simulink library "lib_transmission2"  (Simulink 4.1.1)
values from neighbouring files (symbols this model uses):
  logFlag = 1    [advSACompMaskInit.m]    (also in advSACompMaskInitR13.m)
undefined symbols (not defined in the file or in its folder): cyc_mph, fc_map_spd, fc_max_trq, fc_spd_scale, fc_trq_scale, fd_inertia, fd_loss, fd_ratio, gb_dnshift_load, gb_dnshift_spd, gb_gear_number_lookup, gb_gears_num, gb_inertia, gb_loss_const, gb_loss_input_spd_coeff, gb_loss_input_trq_coeff, gb_loss_output_spd_coeff, gb_loss_output_trq_coeff, gb_map_spd_out, gb_map_trq_in, gb_map_trq_out, gb_num_init, gb_ratio, gb_shift_delay, gb_spd_scale, gb_trq_scale, gb_upshift_load, gb_upshift_spd, htc_inertia, htc_k_adv, htc_k_adv_coast, htc_lockup, htc_lockup_load, htc_lockup_spd, htc_lu_gear_range, htc_max_coast_tr, htc_min_coast_tr, htc_pump_loss_spd, htc_pump_loss_trq_lockup, htc_pump_loss_trq_unlock, htc_sr, htc_sr_coast, htc_tr, htc_tr_coast, htc_unlock_spd, mc_map_spd, mc_max_trq, mc_overtrq_factor, mc_spd_scale, mc_trq_scale, tc_loss, tc_mc_to_fc_ratio, tx_eff_map, tx_map_spd, tx_map_trq, tx_pg_r, tx_pg_s, tx_speed_dep, vc_clutch_bool, vc_idle_spd ... (+2)
libraries: lib_controls x1, lib_etc x1, lib_controls2 x1, lib_transmission x1
(part 12 of 17)

== system lib_transmission2/Gearbox Control/Gearbox Control manual shift logic/manual shift logic/gearbox  control ==
  note: local GOTO blocks:
  gb_trq_out_r : Inport  Port=1  LatchInput=off
  gb_spd_out_r : Inport  Port=2  LatchInput=off
  prev. Pout/Pin : Inport  Port=3  LatchInput=off
  tires are at traction limit : Inport  Port=4  LatchInput=off
  Block NOTES : Subsystem
      settings: RTWFcnNameOpts=Auto  RTWFileNameOpts=Auto
      mask Display: disp('Block\nNOTES')
  Constant : Constant  Orientation=left  Value=1
  Fcn : Fcn  Expr=1/u
  Fcn1 : Fcn  Orientation=up  Expr=1/u
  Gain1 : Gain  Gain=-1  Multiplication=Element-wise(K.*u)  SaturateOnIntegerOverflow=on
  Product2 : Product  Inputs=*/  Multiplication=Element-wise(.*)  SaturateOnIntegerOverflow=on
  Product3 : Product  Inputs=2  Multiplication=Element-wise(.*)  SaturateOnIntegerOverflow=on
  Rate Limiter : RateLimiter  Orientation=left  RisingSlewLimit=1/(gb_shift_delay+eps)  FallingSlewLimit=-1/(gb_shift_delay+eps)
  Saturation : Saturate  UpperLimit=1  LowerLimit=0.2  LinearizeAsGain=on
  Saturation1 : Saturate  UpperLimit=gb_gears_num  LowerLimit=1  LinearizeAsGain=on
  Switch : Switch  Threshold=eps
  allow downshift? : Subsystem
      settings: RTWFcnNameOpts=Auto  RTWFileNameOpts=Auto
  current gear number : Sum  Inputs=++  SaturateOnIntegerOverflow=on
  delta gear number : Switch  Threshold=eps
  downshift  command : Subsystem
      settings: RTWFcnNameOpts=Auto  RTWFileNameOpts=Auto
  engine torque capability : Lookup  Orientation=left  InputValues=fc_map_spd*fc_spd_scale  OutputValues=fc_max_trq*fc_trq_scale+eps
  est eng trq : Sum  Inputs=++  SaturateOnIntegerOverflow=on
  gb_spd_in_r : Product  Inputs=2  Multiplication=Element-wise(.*)  SaturateOnIntegerOverflow=on
  gear ratio : Lookup  Orientation=left  InputValues=[1:length(gb_ratio)]  OutputValues=gb_ratio
  gear ratio1 : Lookup  InputValues=[1:length(gb_ratio)]  OutputValues=gb_ratio
  gearbox speed estimator : Subsystem
      settings: RTWFcnNameOpts=Auto  RTWFileNameOpts=Auto
  load=T/ (maxT at spd) : Saturate  UpperLimit=1  LowerLimit=0  LinearizeAsGain=on
  prev gear number : Memory  Orientation=left  X0=gb_num_init  InheritSampleTime=off
      settings: RTWStateStorageClass=Auto
  prev gear ratio : Memory  Orientation=left  X0=gb_ratio(gb_num_init)  InheritSampleTime=off
      settings: RTWStateStorageClass=Auto
  shifting1 : Subsystem
      settings: RTWFcnNameOpts=Auto  RTWFileNameOpts=Auto
  upshift  command : Subsystem
      settings: RTWFcnNameOpts=Auto  RTWFileNameOpts=Auto
  ~gb_trq_in_r : Product  Inputs=3  Multiplication=Element-wise(.*)  SaturateOnIntegerOverflow=on
  gear ratio2 : Outport  Port=1  InitialOutput=0
  shifting : Outport  Port=2  InitialOutput=0
  gear number : Outport  Port=3  InitialOutput=0
  wires:
  [acc_mech_trq_est] -> est eng trq/2
  shifting1/1(out_1) -> shifting/1
  gear ratio1/1 -> gear ratio2/1
  current gear number/1 -> Saturation1/1
  Saturation/1 -> Fcn/1
  prev. Pout/Pin/1 -> Saturation/1
  gb_trq_out_r/1 -> ~gb_trq_in_r/1
  upshift  command/1(command) -> delta gear number/1, delta gear number/2
  downshift  command/1(command) -> Gain1/1
  Fcn1/1 -> ~gb_trq_in_r/3
  engine torque capability/1 -> Product2/2
  Fcn/1 -> ~gb_trq_in_r/2
  Saturation1/1 -> prev gear number/1, gear ratio1/1, gear number/1, Rate Limiter/1, shifting1/1(gear number)
  prev gear number/1 -> allow downshift?/1(prev gearnum), upshift  command/1(prev gear number), downshift  command/1(prev gear number), current gear number/1
  Product2/1 -> load=T/ (maxT at spd)/1
  Constant/1 -> Switch/1
  tires are at traction limit/1 -> Switch/2
  Rate Limiter/1 -> gear ratio/1
  gb_spd_out_r/1 -> gb_spd_in_r/1
  gb_spd_in_r/1 -> gearbox speed estimator/1(gb_spd_in_r if no gear change)
  gear ratio/1 -> prev gear ratio/1
  prev gear ratio/1 -> gb_spd_in_r/2, Fcn1/1
  Gain1/1 -> Product3/2
  Product3/1 -> delta gear number/3
  allow downshift?/1(allow shift) -> Product3/1
  gearbox speed estimator/1(Out1) -> engine torque capability/1, downshift  command/3(engine speed), upshift  command/3(engine speed)
  ~gb_trq_in_r/1 -> est eng trq/1
  est eng trq/1 -> Product2/1
  load=T/ (maxT at spd)/1 -> Switch/3
  Switch/1 -> upshift  command/2(engine load), downshift  command/2(engine load)
  delta gear number/1 -> current gear number/2

== system lib_transmission2/Gearbox Control/automatic transmission gearbox and htc advanced lock-up logic for htc shift logic for gearbox/gearbox control for use w/ AT/Block NOTES ==
  note: Lock-up of the HTC occurs when it is supposed to for the current gear, AND
      | the transmission isn't shifting, AND
      | the lockup wouldn't precipitate an immediate downshift.
  note: This gearbox control block computes the current gear number given the gearbox's
      | req'd output torque and speed and an estimate its efficiency.  Upshifts occur, given a
      | certain engine speed,  when the estimated engine load falls below the upshift curve
      | in engine speed/load space, and downshifts likewise occur when estimated engine
      | load rises above the downshift curve.  Separate upshift and downshift curves are
      | defined for each gear.  An upshift may not be immediately followed by a downshift.
      | If the tires are about to slip, don't upshift unless the engine would be at max. speed.
      | Enforce this rule by setting the load to 1 when the tires are about to slip.

== system lib_transmission2/Gearbox Control/automatic transmission gearbox and htc advanced lock-up logic for htc shift logic for gearbox/gearbox control for use w/ AT/Speed Dependent Shifting ==
  note: storing shifting and gear ratio
      | information to workspace
  note: decel case
  note: accel case
  note: accel
      | case
  note: decel
      | case
  note: delta speed
  note: SPEED
      | DEPENDENT
      | SHIFT
      | SIGNAL
  "velocity required (limited) " : Inport  Port=1  LatchInput=off
  Look-Up Table (gear for downshift) : Lookup  InputValues="tx_spd_dep_dnshift(:,1)   % vector of speeds m/s"  OutputValues="tx_spd_dep_dnshift(:,2)  % gear number--must be step function"
  Look-Up Table (gear for upshift) : Lookup  InputValues="tx_spd_dep_upshift(:,1)   % vector of speeds in m/s"  OutputValues="tx_spd_dep_upshift(:,2)  % gear number--must be step function"
  Mux : Mux  Inputs=2
      settings: DisplayOption=none
  Mux2 : Mux  Inputs=2
      settings: DisplayOption=none
  New gear ratio : ToWorkspace  VariableName=new_gear_ratio  SampleTime=0  SaveFormat=Array
      settings: MaxDataPoints=50000
  Rounding Function : Rounding  Operator=round
  Rounding Function1 : Rounding  Operator=round
  Saturation4 : Saturate  UpperLimit=gb_gears_num  LowerLimit=1  LinearizeAsGain=on
  Saturation5 : Saturate  UpperLimit=gb_gears_num  LowerLimit=1  LinearizeAsGain=on
  "delta speed (\"+\" is acceleration)" : Sum  Inputs=-+  SaturateOnIntegerOverflow=on
  gear ratio6 : Lookup  InputValues=[1:length(gb_ratio)]  OutputValues=gb_ratio
  gear ratio8 : Lookup  InputValues=[1:length(gb_ratio)]  OutputValues=gb_ratio
  prev veh speed : Memory  X0=1  InheritSampleTime=off
      settings: RTWStateStorageClass=Auto
  shifting : Subsystem  AncestorBlock=lib_controls/SubSystem/shifting
      settings: RTWFcnNameOpts=Auto  RTWFileNameOpts=Auto
  shifting1 : Subsystem  AncestorBlock=lib_controls/SubSystem/shifting
      settings: RTWFcnNameOpts=Auto  RTWFileNameOpts=Auto
  switch for gear number : Switch  Threshold=eps
  switch for gear ratio and shifting (muxed) : Switch  Threshold=eps
  total fuel used (gal) : ToWorkspace  VariableName=neg_gear_num  SampleTime=0  SaveFormat=Array
      settings: MaxDataPoints=50000
  gear ratio and shifting : Outport  Orientation=up  Port=1
  gear number : Outport  Port=2
  wires:
  Rounding Function1/1 -> Saturation5/1
  Look-Up Table (gear for downshift)/1 -> Rounding Function1/1
  Rounding Function/1 -> Saturation4/1
  Look-Up Table (gear for upshift)/1 -> Rounding Function/1
  "delta speed (\"+\" is acceleration)"/1 -> switch for gear ratio and shifting (muxed)/2, switch for gear number/2
  switch for gear number/1 -> gear number/1
  switch for gear ratio and shifting (muxed)/1 -> gear ratio and shifting/1, New gear ratio/1
  Saturation4/1 -> gear ratio6/1, shifting1/1(gear number), switch for gear number/1
  shifting1/1(out_1) -> Mux/2
  gear ratio6/1 -> Mux/1
  Saturation5/1 -> shifting/1(gear number), gear ratio8/1, total fuel used (gal)/1, switch for gear number/3
  gear ratio8/1 -> Mux2/1
  shifting/1(out_1) -> Mux2/2
  Mux/1 -> switch for gear ratio and shifting (muxed)/1
  Mux2/1 -> switch for gear ratio and shifting (muxed)/3
  prev veh speed/1 -> "delta speed (\"+\" is acceleration)"/1
  "velocity required (limited) "/1 -> Look-Up Table (gear for upshift)/1, Look-Up Table (gear for downshift)/1, "delta speed (\"+\" is acceleration)"/2, prev veh speed/1

== system lib_transmission2/Gearbox Control/automatic transmission gearbox and htc advanced lock-up logic for htc shift logic for gearbox/gearbox control for use w/ AT/allow downshift? ==
  prev gearnum : Inport  Port=1  LatchInput=off
  Logical Operator : Logic  Operator=NOR  Inputs=2
  Memory : Memory  X0=1  InheritSampleTime=off
      settings: RTWStateStorageClass=Auto
  Memory1 : Memory  X0=1  InheritSampleTime=off
      settings: RTWStateStorageClass=Auto
  Relational Operator1 : RelationalOperator  Operator=>
  Relational Operator2 : RelationalOperator  Operator=>
  allow shift : Outport  Port=1  InitialOutput=0
  wires:
  Logical Operator/1 -> allow shift/1
  prev gearnum/1 -> Relational Operator1/1, Memory/1, Relational Operator2/1
  Relational Operator1/1 -> Logical Operator/1
  Memory/1 -> Relational Operator1/2, Memory1/1
  Memory1/1 -> Relational Operator2/2
  Relational Operator2/1 -> Logical Operator/2

== system lib_transmission2/Gearbox Control/automatic transmission gearbox and htc advanced lock-up logic for htc shift logic for gearbox/gearbox control for use w/ AT/downshift  command ==
  prev gear number : Inport  Port=1  LatchInput=off
  engine load : Inport  Port=2  LatchInput=off
  engine speed : Inport  Port=3  LatchInput=off
  Mux : Mux  Inputs=2
      settings: DisplayOption=none
  Relational Operator : RelationalOperator  Operator=>
  load fraction : Subsystem  mask(Gear Selector){spd=gb_dnshift_spd, load=gb_dnshift_load}
      mask prompts: spd "Speeds:"; load "Load Fractions:"
      mask help:
      | This block will perform a linear interplation (extrapolation outside of bounds) to determine the shift point load fraction associated with the current gear number and speed.
      |
      | The Speeds parameter should be defined as an array of vectors containing speeds for each gear number.  The Load Fractions parameter should be defined as a array of vectors containing load fractions indexed by the speeds in the Speeds parameter for each gear number.
      settings: RTWFcnNameOpts=Auto  RTWFileNameOpts=Auto
      mask Help:
      | Reference the base workspace variables - gb_**shift_spd and gb_**shift_load  where ** is either up for upshift conditions or dn for downshift conditions.
      | 
      | Or define the arrays as follows:
      | 
      | {[spd1 spd2 spd3 spd4]; [spd1 spd2 spd3 spd4]; ...}
      | 
      | {[load1 load2 load3 load4]; [load1 load2 load3 load4]; ...}
      | 
      | where each array contains one row for each gear in the gearbox.  Speeds should be defined in rad/s and loads as a decimal fraction.
  command : Outport  Port=1  InitialOutput=0
  wires:
  Relational Operator/1 -> command/1
  engine speed/1 -> Mux/2
  prev gear number/1 -> Mux/1
  engine load/1 -> Relational Operator/1
  Mux/1 -> load fraction/1(In1)
  load fraction/1(Out1) -> Relational Operator/2

== system lib_transmission2/Gearbox Control/automatic transmission gearbox and htc advanced lock-up logic for htc shift logic for gearbox/gearbox control for use w/ AT/downshift  command1 ==
  prev gear number : Inport  Port=1  LatchInput=off
  engine load : Inport  Port=2  LatchInput=off
  engine speed : Inport  Port=3  LatchInput=off
  Mux : Mux  Inputs=2
      settings: DisplayOption=none
  Relational Operator : RelationalOperator  Operator=>
  load fraction : Subsystem  mask(Gear Selector){spd=gb_dnshift_spd, load=gb_dnshift_load}
      mask prompts: spd "Speeds:"; load "Load Fractions:"
      mask help:
      | This block will perform a linear interplation (extrapolation outside of bounds) to determine the shift point load fraction associated with the current gear number and speed.
      |
      | The Speeds parameter should be defined as an array of vectors containing speeds for each gear number.  The Load Fractions parameter should be defined as a array of vectors containing load fractions indexed by the speeds in the Speeds parameter for each gear number.
      settings: RTWFcnNameOpts=Auto  RTWFileNameOpts=Auto
      mask Help:
      | Reference the base workspace variables - gb_**shift_spd and gb_**shift_load  where ** is either up for upshift conditions or dn for downshift conditions.
      | 
      | Or define the arrays as follows:
      | 
      | {[spd1 spd2 spd3 spd4]; [spd1 spd2 spd3 spd4]; ...}
      | 
      | {[load1 load2 load3 load4]; [load1 load2 load3 load4]; ...}
      | 
      | where each array contains one row for each gear in the gearbox.  Speeds should be defined in rad/s and loads as a decimal fraction.
  command : Outport  Port=1  InitialOutput=0
  wires:
  engine speed/1 -> Mux/2
  load fraction/1(Out1) -> Relational Operator/2
  Mux/1 -> load fraction/1(In1)
  engine load/1 -> Relational Operator/1
  prev gear number/1 -> Mux/1
  Relational Operator/1 -> command/1

== system lib_transmission2/Gearbox Control/automatic transmission gearbox and htc advanced lock-up logic for htc shift logic for gearbox/gearbox control for use w/ AT/est. engine trq and spd ==
  prev gear number : Inport  Port=1  LatchInput=off
  " prev eta_gb" : Inport  Port=2  LatchInput=off
  gb_trq_out_r : Inport  Port=3  LatchInput=off
  gb_spd_out_r : Inport  Port=4  LatchInput=off
  Block NOTES : Subsystem
      settings: RTWFcnNameOpts=Auto  RTWFileNameOpts=Auto
      mask Display: disp('Block\nNOTES')
  Constant2 : Constant  Orientation=left  Value=[1 1]
  Constant5 : Constant  Orientation=left  Value=0
  Demux : Demux  Outputs=2  BusSelectionMode=off
  K_adv : Subsystem
      settings: RTWFcnNameOpts=Auto  RTWFileNameOpts=Auto
  Logical Operator : Logic  Operator=AND  Inputs=2
  Logical Operator1 : Logic  Operator=NOT  Inputs=1
  Memory : Memory  X0=0  InheritSampleTime=off
      settings: RTWStateStorageClass=Auto
  Mux1 : Mux  Inputs=2
      settings: DisplayOption=none
  Mux2 : Mux  Inputs=2
      settings: DisplayOption=none
  Relational Operator1 : RelationalOperator  Operator=>
  SR Look-Up Table SR=wout/win : Lookup  InputValues=htc_k_adv  OutputValues=htc_sr
  Saturation1 : Saturate  UpperLimit=1  LowerLimit=0.7  LinearizeAsGain=on
  Saturation2 : Saturate  UpperLimit=inf  LowerLimit=0  LinearizeAsGain=on
  Switch : Switch  Threshold=eps
  TR Look-Up Table TR=Tout/Tin : Lookup  InputValues=htc_k_adv  OutputValues=htc_tr
  TR,SR : Mux  Inputs=2
      settings: DisplayOption=none
  est eng trq : Sum  Inputs=++  SaturateOnIntegerOverflow=on
  gear ratio1 : Lookup  InputValues=[1:length(gb_ratio)]  OutputValues=gb_ratio
  ~eng trq and spd : Product  Inputs=*/  Multiplication=Element-wise(.*)  SaturateOnIntegerOverflow=on
  ~gb_spd_in_r : Product  Inputs=2  Multiplication=Element-wise(.*)  SaturateOnIntegerOverflow=on
  ~gb_trq_in_r : Product  Inputs=//*  Multiplication=Element-wise(.*)  SaturateOnIntegerOverflow=on
  est eng trq (Nm) : Outport  Port=1
  est eng spd (rad/s) : Outport  Port=2
  gb_spd_in_est (rad/s)1 : Outport  Port=3
  wires:
  est eng trq/1 -> Mux1/1, Relational Operator1/1, Mux2/1
  ~gb_trq_in_r/1 -> est eng trq/1
  ~gb_spd_in_r/1 -> Mux2/2, gb_spd_in_est (rad/s)1/1, Mux1/2
  [acc_mech_trq_est] -> est eng trq/2
  SR Look-Up Table SR=wout/win/1 -> TR,SR/2
  TR Look-Up Table TR=Tout/Tin/1 -> TR,SR/1
  K_adv/1(K_adv) -> SR Look-Up Table SR=wout/win/1, TR Look-Up Table TR=Tout/Tin/1
  Mux2/1 -> K_adv/1("Req'd output trq and spd (Nm), (rad/s)")
  ~eng trq and spd/1 -> Demux/1
  Mux1/1 -> ~eng trq and spd/1
  [locked_up] -> Memory/1
  Logical Operator/1 -> Switch/2
  Logical Operator1/1 -> Logical Operator/2
  Memory/1 -> Logical Operator1/1
  Demux/1 -> est eng trq (Nm)/1
  prev gear number/1 -> gear ratio1/1
  Relational Operator1/1 -> Logical Operator/1
  Constant5/1 -> Relational Operator1/2
  Saturation2/1 -> est eng spd (rad/s)/1
  Demux/2 -> Saturation2/1
  Saturation1/1 -> ~gb_trq_in_r/2
  " prev eta_gb"/1 -> Saturation1/1
  Switch/1 -> ~eng trq and spd/2
  Constant2/1 -> Switch/3
  TR,SR/1 -> Switch/1
  gear ratio1/1 -> ~gb_spd_in_r/1, ~gb_trq_in_r/1
  gb_spd_out_r/1 -> ~gb_spd_in_r/2
  gb_trq_out_r/1 -> ~gb_trq_in_r/3

== system lib_transmission2/Gearbox Control/automatic transmission gearbox and htc advanced lock-up logic for htc shift logic for gearbox/gearbox control for use w/ AT/est. engine trq and spd assuming lockup ==
  new gear number : Inport  Port=1  LatchInput=off
  " prev eta_gb" : Inport  Port=2  LatchInput=off
  gb_trq_out_r : Inport  Port=3  LatchInput=off
  gb_spd_in_est : Inport  Port=4  LatchInput=off
  Block NOTES : Subsystem
      settings: RTWFcnNameOpts=Auto  RTWFileNameOpts=Auto
      mask Display: disp('Block\nNOTES')
  Memory : Memory  X0=gb_ratio(1)  InheritSampleTime=off
      settings: RTWStateStorageClass=Auto
  Saturation1 : Saturate  UpperLimit=1  LowerLimit=0.7  LinearizeAsGain=on
  Saturation2 : Saturate  UpperLimit=inf  LowerLimit=0  LinearizeAsGain=on
  est eng trq : Sum  Inputs=++  SaturateOnIntegerOverflow=on
  gear ratio1 : Lookup  InputValues=[1:length(gb_ratio)]  OutputValues=gb_ratio
  ~gb_spd_in_r : Product  Inputs=*/*  Multiplication=Element-wise(.*)  SaturateOnIntegerOverflow=on
  ~gb_trq_in_r : Product  Inputs=//*  Multiplication=Element-wise(.*)  SaturateOnIntegerOverflow=on
  est eng trq (Nm) : Outport  Port=1
  est eng spd (rad/s) : Outport  Port=2
  wires:
  ~gb_spd_in_r/1 -> Saturation2/1
  est eng trq/1 -> est eng trq (Nm)/1
  ~gb_trq_in_r/1 -> est eng trq/1
  [acc_mech_trq_est] -> est eng trq/2
  gb_spd_in_est/1 -> ~gb_spd_in_r/3
  Memory/1 -> ~gb_spd_in_r/2
  Saturation2/1 -> est eng spd (rad/s)/1
  new gear number/1 -> gear ratio1/1
  gb_trq_out_r/1 -> ~gb_trq_in_r/3
  gear ratio1/1 -> Memory/1, ~gb_spd_in_r/1, ~gb_trq_in_r/1
  " prev eta_gb"/1 -> Saturation1/1
  Saturation1/1 -> ~gb_trq_in_r/2

== system lib_transmission2/Gearbox Control/automatic transmission gearbox and htc advanced lock-up logic for htc shift logic for gearbox/gearbox control for use w/ AT/htc lockup logic ==
  engine load (%) : Inport  Port=1  LatchInput=off
  gear num : Inport  Port=2  LatchInput=off
  Constant1 : Constant  Orientation=left  Value=0.5
  Constant2 : Constant  Value=0
  Constant3 : Constant  Value=0
  Constant4 : Constant  Value=-1
  Logical Operator : Logic  Operator=NOR  Inputs=2
  Memory1 : Memory  Orientation=left  X0=1  InheritSampleTime=off
      settings: RTWStateStorageClass=Auto
  Memory2 : Memory  X0=1  InheritSampleTime=off
      settings: RTWStateStorageClass=Auto
  Memory3 : Memory  X0=1  InheritSampleTime=off
      settings: RTWStateStorageClass=Auto
  Relational Operator : RelationalOperator  Operator=>=
  Relational Operator1 : RelationalOperator  Operator=>
  Relational Operator2 : RelationalOperator  Operator=<
  Relational Operator3 : RelationalOperator  Operator=<
  Saturation1 : Saturate  UpperLimit=1  LowerLimit=0  LinearizeAsGain=on
  Switch{,1..3} (4 alike) : Switch  Threshold=0.5
  current lock/unlock  status : Sum  Inputs=++  SaturateOnIntegerOverflow=on
  lock-up in high gears : Lookup  InputValues=[1:length(htc_lockup)]  OutputValues=htc_lockup
  lock-up in this gear : Lookup  InputValues=htc_lockup_load  OutputValues=htc_lockup_spd
  lock/unlock  gear range : Lookup  InputValues=[1:length(htc_lockup)]  OutputValues=htc_lu_gear_range
  unlock in this gear : Lookup  InputValues=htc_lockup_load  OutputValues=htc_unlock_spd
  htc L/UL : Outport  Port=1
  wires:
  Constant1/1 -> Relational Operator/2, Relational Operator1/1
  gear num/1 -> lock-up in high gears/1, lock/unlock  gear range/1
  lock-up in high gears/1 -> Relational Operator/1
  Relational Operator/1 -> Switch/2, Switch/1
  Switch/1 -> htc L/UL/1, Memory1/1
  lock/unlock  gear range/1 -> Relational Operator1/2
  lock-up in this gear/1 -> Relational Operator2/1
  unlock in this gear/1 -> Relational Operator3/2
  Relational Operator1/1 -> Switch1/2
  Constant2/1 -> Switch1/1
  Switch1/1 -> Switch/3
  Saturation1/1 -> Switch1/3
  Relational Operator2/1 -> Logical Operator/1, Switch3/2, Switch3/1
  Relational Operator3/1 -> Logical Operator/2
  Logical Operator/1 -> Switch2/2
  Constant3/1 -> Switch2/3
  Switch3/1 -> Switch2/1
  Constant4/1 -> Switch3/3
  current lock/unlock  status/1 -> Saturation1/1
  Memory1/1 -> current lock/unlock  status/1
  Switch2/1 -> current lock/unlock  status/2
  Memory2/1 -> Relational Operator2/2, Relational Operator3/1
  Memory3/1 -> lock-up in this gear/1, unlock in this gear/1
  engine load (%)/1 -> Memory3/1
  [gb_trq_out_a] -> Memory2/1

== system lib_transmission2/Gearbox Control/automatic transmission gearbox and htc advanced lock-up logic for htc shift logic for gearbox/gearbox control for use w/ AT/shifting1 ==
  gear number : Inport  Port=1  LatchInput=off
  Constant : Constant  Value=gb_shift_delay-1e-6
  Relational Operator : RelationalOperator  Operator=<
  time since last shift : Subsystem
      settings: RTWFcnNameOpts=Auto  RTWFileNameOpts=Auto
      mask Display: disp('time since\nlast shift')
  out_1 : Outport  Port=1  InitialOutput=0
  wires:
  Relational Operator/1 -> out_1/1
  gear number/1 -> time since last shift/1(in_1)
  Constant/1 -> Relational Operator/2
  time since last shift/1(out_1) -> Relational Operator/1

== system lib_transmission2/Gearbox Control/automatic transmission gearbox and htc advanced lock-up logic for htc shift logic for gearbox/gearbox control for use w/ AT/upshift  command ==
  prev gear number : Inport  Port=1  LatchInput=off
  engine load : Inport  Port=2  LatchInput=off
  engine speed : Inport  Port=3  LatchInput=off
  Mux : Mux  Inputs=2
      settings: DisplayOption=none
  Relational Operator : RelationalOperator  Operator=<
  load fraction : Subsystem  mask(Gear Selector){spd=gb_upshift_spd, load=gb_upshift_load}
      mask prompts: spd "Speeds:"; load "Load Fractions:"
      mask help:
      | This block will perform a linear interplation (extrapolation outside of bounds) to determine the shift point load fraction associated with the current gear number and speed.
      |
      | The Speeds parameter should be defined as an array of vectors containing speeds for each gear number.  The Load Fractions parameter should be defined as a array of vectors containing load fractions indexed by the speeds in the Speeds parameter for each gear number.
      settings: RTWFcnNameOpts=Auto  RTWFileNameOpts=Auto
      mask Help:
      | Reference the base workspace variables - gb_**shift_spd and gb_**shift_load  where ** is either up for upshift conditions or dn for downshift conditions.
      | 
      | Or define the arrays as follows:
      | 
      | {[spd1 spd2 spd3 spd4]; [spd1 spd2 spd3 spd4]; ...}
      | 
      | {[load1 load2 load3 load4]; [load1 load2 load3 load4]; ...}
      | 
      | where each array contains one row for each gear in the gearbox.  Speeds should be defined in rad/s and loads as a decimal fraction.
  command : Outport  Port=1  InitialOutput=0
  wires:
  Relational Operator/1 -> command/1
  engine speed/1 -> Mux/2
  Mux/1 -> load fraction/1(In1)
  prev gear number/1 -> Mux/1
  engine load/1 -> Relational Operator/1
  load fraction/1(Out1) -> Relational Operator/2

== system lib_transmission2/Gearbox Control/automatic transmission gearbox and htc standard lockup logic for htc shift logic for gearbox/gearbox control for use w/ AT/Block NOTES ==
  note: This gearbox control block computes the current gear number given the gearbox's
      | req'd output torque and speed and an estimate its efficiency.  Upshifts occur, given a
      | certain engine speed,  when the estimated engine load falls below the upshift curve
      | in engine speed/load space, and downshifts likewise occur when estimated engine
      | load rises above the downshift curve.  Separate upshift and downshift curves are
      | defined for each gear.  An upshift may not be immediately followed by a downshift.
      | If the tires are about to slip, don't upshift unless the engine would be at max. speed.
      | Enforce this rule by setting the load to 1 when the tires are about to slip.
  note: Lock-up of the HTC occurs when it is supposed to for the current gear, AND
      | the transmission isn't shifting, AND
      | the lockup wouldn't precipitate an immediate downshift.

== system lib_transmission2/Gearbox Control/automatic transmission gearbox and htc standard lockup logic for htc shift logic for gearbox/gearbox control for use w/ AT/allow downshift? ==
  prev gearnum : Inport  Port=1  LatchInput=off
  Logical Operator : Logic  Operator=NOR  Inputs=2
  Memory : Memory  X0=1  InheritSampleTime=off
      settings: RTWStateStorageClass=Auto
  Memory1 : Memory  X0=1  InheritSampleTime=off
      settings: RTWStateStorageClass=Auto
  Relational Operator1 : RelationalOperator  Operator=>
  Relational Operator2 : RelationalOperator  Operator=>
  allow shift : Outport  Port=1  InitialOutput=0
  wires:
  Relational Operator2/1 -> Logical Operator/2
  Memory1/1 -> Relational Operator2/2
  Memory/1 -> Memory1/1, Relational Operator1/2
  Relational Operator1/1 -> Logical Operator/1
  prev gearnum/1 -> Relational Operator2/1, Memory/1, Relational Operator1/1
  Logical Operator/1 -> allow shift/1

== system lib_transmission2/Gearbox Control/automatic transmission gearbox and htc standard lockup logic for htc shift logic for gearbox/gearbox control for use w/ AT/downshift  command ==
  prev gear number : Inport  Port=1  LatchInput=off
  engine load : Inport  Port=2  LatchInput=off
  engine speed : Inport  Port=3  LatchInput=off
  Mux : Mux  Inputs=2
      settings: DisplayOption=none
  Relational Operator : RelationalOperator  Operator=>
  load fraction : Subsystem  mask(Gear Selector){spd=gb_dnshift_spd, load=gb_dnshift_load}
      mask prompts: spd "Speeds:"; load "Load Fractions:"
      mask help:
      | This block will perform a linear interplation (extrapolation outside of bounds) to determine the shift point load fraction associated with the current gear number and speed.
      |
      | The Speeds parameter should be defined as an array of vectors containing speeds for each gear number.  The Load Fractions parameter should be defined as a array of vectors containing load fractions indexed by the speeds in the Speeds parameter for each gear number.
      settings: RTWFcnNameOpts=Auto  RTWFileNameOpts=Auto
      mask Help:
      | Reference the base workspace variables - gb_**shift_spd and gb_**shift_load  where ** is either up for upshift conditions or dn for downshift conditions.
      | 
      | Or define the arrays as follows:
      | 
      | {[spd1 spd2 spd3 spd4]; [spd1 spd2 spd3 spd4]; ...}
      | 
      | {[load1 load2 load3 load4]; [load1 load2 load3 load4]; ...}
      | 
      | where each array contains one row for each gear in the gearbox.  Speeds should be defined in rad/s and loads as a decimal fraction.
  command : Outport  Port=1  InitialOutput=0
  wires:
  load fraction/1(Out1) -> Relational Operator/2
  Mux/1 -> load fraction/1(In1)
  engine load/1 -> Relational Operator/1
  prev gear number/1 -> Mux/1
  engine speed/1 -> Mux/2
  Relational Operator/1 -> command/1

== system lib_transmission2/Gearbox Control/automatic transmission gearbox and htc standard lockup logic for htc shift logic for gearbox/gearbox control for use w/ AT/downshift  command1 ==
  prev gear number : Inport  Port=1  LatchInput=off
  engine load : Inport  Port=2  LatchInput=off
  engine speed : Inport  Port=3  LatchInput=off
  Mux : Mux  Inputs=2
      settings: DisplayOption=none
  Relational Operator : RelationalOperator  Operator=>
  load fraction : Subsystem  mask(Gear Selector){spd=gb_dnshift_spd, load=gb_dnshift_load}
      mask prompts: spd "Speeds:"; load "Load Fractions:"
      mask help:
      | This block will perform a linear interplation (extrapolation outside of bounds) to determine the shift point load fraction associated with the current gear number and speed.
      |
      | The Speeds parameter should be defined as an array of vectors containing speeds for each gear number.  The Load Fractions parameter should be defined as a array of vectors containing load fractions indexed by the speeds in the Speeds parameter for each gear number.
      settings: RTWFcnNameOpts=Auto  RTWFileNameOpts=Auto
      mask Help:
      | Reference the base workspace variables - gb_**shift_spd and gb_**shift_load  where ** is either up for upshift conditions or dn for downshift conditions.
      | 
      | Or define the arrays as follows:
      | 
      | {[spd1 spd2 spd3 spd4]; [spd1 spd2 spd3 spd4]; ...}
      | 
      | {[load1 load2 load3 load4]; [load1 load2 load3 load4]; ...}
      | 
      | where each array contains one row for each gear in the gearbox.  Speeds should be defined in rad/s and loads as a decimal fraction.
  command : Outport  Port=1  InitialOutput=0
  wires:
  Relational Operator/1 -> command/1
  prev gear number/1 -> Mux/1
  engine load/1 -> Relational Operator/1
  Mux/1 -> load fraction/1(In1)
  load fraction/1(Out1) -> Relational Operator/2
  engine speed/1 -> Mux/2

== system lib_transmission2/Gearbox Control/automatic transmission gearbox and htc standard lockup logic for htc shift logic for gearbox/gearbox control for use w/ AT/est. engine trq and spd ==
  prev gear number : Inport  Port=1  LatchInput=off
  " prev eta_gb" : Inport  Port=2  LatchInput=off
  gb_trq_out_r : Inport  Port=3  LatchInput=off
  gb_spd_out_r : Inport  Port=4  LatchInput=off
  Block NOTES : Subsystem
      settings: RTWFcnNameOpts=Auto  RTWFileNameOpts=Auto
      mask Display: disp('Block\nNOTES')
  Constant2 : Constant  Orientation=left  Value=[1 1]
  Constant5 : Constant  Orientation=left  Value=0
  Demux : Demux  Outputs=2  BusSelectionMode=off
  K_adv : Subsystem
      settings: RTWFcnNameOpts=Auto  RTWFileNameOpts=Auto
  Logical Operator : Logic  Operator=AND  Inputs=2
  Logical Operator1 : Logic  Operator=NOT  Inputs=1
  Mux1 : Mux  Inputs=2
      settings: DisplayOption=none
  Mux2 : Mux  Inputs=2
      settings: DisplayOption=none
  Relational Operator1 : RelationalOperator  Operator=>
  SR Look-Up Table SR=wout/win : Lookup  InputValues=htc_k_adv  OutputValues=htc_sr
  Saturation1 : Saturate  UpperLimit=1  LowerLimit=0.7  LinearizeAsGain=on
  Saturation2 : Saturate  UpperLimit=inf  LowerLimit=0  LinearizeAsGain=on
  Switch : Switch  Threshold=eps
  TR Look-Up Table TR=Tout/Tin : Lookup  InputValues=htc_k_adv  OutputValues=htc_tr
  TR,SR : Mux  Inputs=2
      settings: DisplayOption=none
  est eng trq : Sum  Inputs=++  SaturateOnIntegerOverflow=on
  gear ratio : Lookup  InputValues=[1:length(gb_ratio)]  OutputValues=gb_ratio
  ~eng trq and spd : Product  Inputs=*/  Multiplication=Element-wise(.*)  SaturateOnIntegerOverflow=on
  ~gb_spd_in_r : Product  Inputs=2  Multiplication=Element-wise(.*)  SaturateOnIntegerOverflow=on
  ~gb_trq_in_r : Product  Inputs=//*  Multiplication=Element-wise(.*)  SaturateOnIntegerOverflow=on
  est eng trq (Nm) : Outport  Port=1
  est eng spd (rad/s) : Outport  Port=2
  gb_spd_in_est (rad/s) : Outport  Port=3
  wires:
  gb_trq_out_r/1 -> ~gb_trq_in_r/3
  gb_spd_out_r/1 -> ~gb_spd_in_r/2
  gear ratio/1 -> ~gb_trq_in_r/1, ~gb_spd_in_r/1
  TR,SR/1 -> Switch/1
  Constant2/1 -> Switch/3
  Switch/1 -> ~eng trq and spd/2
  " prev eta_gb"/1 -> Saturation1/1
  Saturation1/1 -> ~gb_trq_in_r/2
  Demux/2 -> Saturation2/1
  Saturation2/1 -> est eng spd (rad/s)/1
  Constant5/1 -> Relational Operator1/2
  Relational Operator1/1 -> Logical Operator/1
  prev gear number/1 -> gear ratio/1
  Demux/1 -> est eng trq (Nm)/1
  Logical Operator1/1 -> Logical Operator/2
  Logical Operator/1 -> Switch/2
  [locked_up_last] -> Logical Operator1/1
  Mux1/1 -> ~eng trq and spd/1
  ~eng trq and spd/1 -> Demux/1
  Mux2/1 -> K_adv/1("Req'd output trq and spd (Nm), (rad/s)")
  K_adv/1(K_adv) -> TR Look-Up Table TR=Tout/Tin/1, SR Look-Up Table SR=wout/win/1
  TR Look-Up Table TR=Tout/Tin/1 -> TR,SR/1
  SR Look-Up Table SR=wout/win/1 -> TR,SR/2
  [acc_mech_trq_est] -> est eng trq/2
  ~gb_spd_in_r/1 -> Mux1/2, gb_spd_in_est (rad/s)/1, Mux2/2
  ~gb_trq_in_r/1 -> est eng trq/1
  est eng trq/1 -> Mux2/1, Relational Operator1/1, Mux1/1

== system lib_transmission2/Gearbox Control/automatic transmission gearbox and htc standard lockup logic for htc shift logic for gearbox/gearbox control for use w/ AT/est. engine trq and spd assuming lockup ==
  new gear number : Inport  Port=1  LatchInput=off
  " prev eta_gb" : Inport  Port=2  LatchInput=off
  gb_trq_out_r : Inport  Port=3  LatchInput=off
  gb_spd_in_est : Inport  Port=4  LatchInput=off
  Block NOTES : Subsystem
      settings: RTWFcnNameOpts=Auto  RTWFileNameOpts=Auto
      mask Display: disp('Block\nNOTES')
  Memory : Memory  X0=gb_ratio(1)  InheritSampleTime=off
      settings: RTWStateStorageClass=Auto
  Saturation1 : Saturate  UpperLimit=1  LowerLimit=0.7  LinearizeAsGain=on
  Saturation2 : Saturate  UpperLimit=inf  LowerLimit=0  LinearizeAsGain=on
  est eng trq : Sum  Inputs=++  SaturateOnIntegerOverflow=on
  gear ratio1 : Lookup  InputValues=[1:length(gb_ratio)]  OutputValues=gb_ratio
  ~gb_spd_in_r : Product  Inputs=*/*  Multiplication=Element-wise(.*)  SaturateOnIntegerOverflow=on
  ~gb_trq_in_r : Product  Inputs=//*  Multiplication=Element-wise(.*)  SaturateOnIntegerOverflow=on
  est eng trq (Nm) : Outport  Port=1
  est eng spd (rad/s) : Outport  Port=2
  wires:
  Saturation1/1 -> ~gb_trq_in_r/2
  " prev eta_gb"/1 -> Saturation1/1
  gear ratio1/1 -> ~gb_trq_in_r/1, ~gb_spd_in_r/1, Memory/1
  gb_trq_out_r/1 -> ~gb_trq_in_r/3
  new gear number/1 -> gear ratio1/1
  Saturation2/1 -> est eng spd (rad/s)/1
  Memory/1 -> ~gb_spd_in_r/2
  gb_spd_in_est/1 -> ~gb_spd_in_r/3
  [acc_mech_trq_est] -> est eng trq/2
  ~gb_trq_in_r/1 -> est eng trq/1
  est eng trq/1 -> est eng trq (Nm)/1
  ~gb_spd_in_r/1 -> Saturation2/1

== system lib_transmission2/Gearbox Control/automatic transmission gearbox and htc standard lockup logic for htc shift logic for gearbox/gearbox control for use w/ AT/shifting1 ==
  gear number : Inport  Port=1  LatchInput=off
  Constant : Constant  Value=gb_shift_delay-1e-6
  Relational Operator : RelationalOperator  Operator=<
  time since last shift : Subsystem
      settings: RTWFcnNameOpts=Auto  RTWFileNameOpts=Auto
      mask Display: disp('time since\nlast shift')
  out_1 : Outport  Port=1  InitialOutput=0
  wires:
  time since last shift/1(out_1) -> Relational Operator/1
  Constant/1 -> Relational Operator/2
  gear number/1 -> time since last shift/1(in_1)
  Relational Operator/1 -> out_1/1

== system lib_transmission2/Gearbox Control/automatic transmission gearbox and htc standard lockup logic for htc shift logic for gearbox/gearbox control for use w/ AT/upshift  command ==
  prev gear number : Inport  Port=1  LatchInput=off
  engine load : Inport  Port=2  LatchInput=off
  engine speed : Inport  Port=3  LatchInput=off
  Mux : Mux  Inputs=2
      settings: DisplayOption=none
  Relational Operator : RelationalOperator  Operator=<
  load fraction : Subsystem  mask(Gear Selector){spd=gb_upshift_spd, load=gb_upshift_load}
      mask prompts: spd "Speeds:"; load "Load Fractions:"
      mask help:
      | This block will perform a linear interplation (extrapolation outside of bounds) to determine the shift point load fraction associated with the current gear number and speed.
      |
      | The Speeds parameter should be defined as an array of vectors containing speeds for each gear number.  The Load Fractions parameter should be defined as a array of vectors containing load fractions indexed by the speeds in the Speeds parameter for each gear number.
      settings: RTWFcnNameOpts=Auto  RTWFileNameOpts=Auto
      mask Help:
      | Reference the base workspace variables - gb_**shift_spd and gb_**shift_load  where ** is either up for upshift conditions or dn for downshift conditions.
      | 
      | Or define the arrays as follows:
      | 
      | {[spd1 spd2 spd3 spd4]; [spd1 spd2 spd3 spd4]; ...}
      | 
      | {[load1 load2 load3 load4]; [load1 load2 load3 load4]; ...}
      | 
      | where each array contains one row for each gear in the gearbox.  Speeds should be defined in rad/s and loads as a decimal fraction.
  command : Outport  Port=1  InitialOutput=0
  wires:
  load fraction/1(Out1) -> Relational Operator/2
  engine load/1 -> Relational Operator/1
  prev gear number/1 -> Mux/1
  Mux/1 -> load fraction/1(In1)
  engine speed/1 -> Mux/2
  Relational Operator/1 -> command/1

== system lib_transmission2/Gearbox Control/time lookup shift logic for gearbox/lookup/shifting determination ==
  gear number : Inport  Port=1  LatchInput=off
  Constant : Constant  Value=gb_shift_delay-1e-6
  Relational Operator : RelationalOperator  Operator=<
  time since last shift : Subsystem
      settings: RTWFcnNameOpts=Auto  RTWFileNameOpts=Auto
      mask Display: disp('time since\nlast shift')
  out_1 : Outport  Port=1  InitialOutput=0
  wires:
  time since last shift/1(out_1) -> Relational Operator/1
  Constant/1 -> Relational Operator/2
  gear number/1 -> time since last shift/1(in_1)
  Relational Operator/1 -> out_1/1

== system lib_transmission2/Gearbox Control/vehicle speed dependent shift logic for gearbox/speed dependent/Speed Dependent Shifting ==
  note: storing shifting and gear ratio
      | information to workspace
  note: decel case
  note: accel case
  note: accel
      | case
  note: decel
      | case
  note: delta speed
  note: SPEED
      | DEPENDENT
      | SHIFT
      | SIGNAL
  "velocity required (limited) " : Inport  Port=1  LatchInput=off
  Look-Up Table (gear for downshift) : Lookup  InputValues="tx_spd_dep_dnshift(:,1)   % vector of speeds m/s"  OutputValues="tx_spd_dep_dnshift(:,2)  % gear number--must be step function"
  Look-Up Table (gear for upshift) : Lookup  InputValues="tx_spd_dep_upshift(:,1)   % vector of speeds in m/s"  OutputValues="tx_spd_dep_upshift(:,2)  % gear number--must be step function"
  Mux : Mux  Inputs=2
      settings: DisplayOption=none
  Mux2 : Mux  Inputs=2
      settings: DisplayOption=none
  New gear ratio : ToWorkspace  VariableName=new_gear_ratio  SampleTime=0  SaveFormat=Array
      settings: MaxDataPoints=50000
  Rounding Function : Rounding  Operator=round
  Rounding Function1 : Rounding  Operator=round
  Saturation4 : Saturate  UpperLimit=gb_gears_num  LowerLimit=1  LinearizeAsGain=on
  Saturation5 : Saturate  UpperLimit=gb_gears_num  LowerLimit=1  LinearizeAsGain=on
  "delta speed (\"+\" is acceleration)" : Sum  Inputs=-+  SaturateOnIntegerOverflow=on
  gear ratio6 : Lookup  InputValues=[1:length(gb_ratio)]  OutputValues=gb_ratio
  gear ratio8 : Lookup  InputValues=[1:length(gb_ratio)]  OutputValues=gb_ratio
  prev veh speed : Memory  X0=1  InheritSampleTime=off
      settings: RTWStateStorageClass=Auto
  shifting : Subsystem
      settings: RTWFcnNameOpts=Auto  RTWFileNameOpts=Auto
  shifting1 : Subsystem
      settings: RTWFcnNameOpts=Auto  RTWFileNameOpts=Auto
  switch for gear number : Switch  Threshold=eps
  switch for gear ratio and shifting (muxed) : Switch  Threshold=eps
  total fuel used (gal) : ToWorkspace  VariableName=neg_gear_num  SampleTime=0  SaveFormat=Array
      settings: MaxDataPoints=50000
  gear ratio and shifting : Outport  Orientation=up  Port=1
  gear number : Outport  Port=2
  wires:
  Rounding Function1/1 -> Saturation5/1
  Look-Up Table (gear for downshift)/1 -> Rounding Function1/1
  Rounding Function/1 -> Saturation4/1
  Look-Up Table (gear for upshift)/1 -> Rounding Function/1
  "delta speed (\"+\" is acceleration)"/1 -> switch for gear ratio and shifting (muxed)/2, switch for gear number/2
  switch for gear number/1 -> gear number/1
  switch for gear ratio and shifting (muxed)/1 -> gear ratio and shifting/1, New gear ratio/1
  Saturation4/1 -> gear ratio6/1, shifting1/1(gear number), switch for gear number/1
  shifting1/1(out_1) -> Mux/2
  gear ratio6/1 -> Mux/1
  Saturation5/1 -> shifting/1(gear number), gear ratio8/1, total fuel used (gal)/1, switch for gear number/3
  gear ratio8/1 -> Mux2/1
  shifting/1(out_1) -> Mux2/2
  Mux/1 -> switch for gear ratio and shifting (muxed)/1
  Mux2/1 -> switch for gear ratio and shifting (muxed)/3
  prev veh speed/1 -> "delta speed (\"+\" is acceleration)"/1
  "velocity required (limited) "/1 -> Look-Up Table (gear for upshift)/1, Look-Up Table (gear for downshift)/1, "delta speed (\"+\" is acceleration)"/2, prev veh speed/1

== system lib_transmission2/clutch <cl>/clutch model and interface/clutch model/Adjust for Possible Launch Speed Request ==
  note: If the clutch is disengaged, under certain
      | circumstances, we will want to request that
      | the input speed to the clutch be ramped up to a
      | given launch speed (decided by the controller)
      | so that the clutch can subsequently slip and
      | engage with a more realistic speed matching
  Input Speed Request : Inport  Port=1  LatchInput=off
  Constant6 : Constant  Value=1
  Logical Operator : Logic  Operator=AND  Inputs=2
  Switch4 : Switch  Threshold=0.5
  clutch disengaged : RelationalOperator  Operator===
  Input Speed Request Adjusted for Launch Speed : Outport  Port=1
  wires:
  [launch_speed] -> Switch4/1
  Switch4/1 -> Input Speed Request Adjusted for Launch Speed/1
  Input Speed Request/1 -> Switch4/3
  [clutch_state] -> clutch disengaged/1
  Constant6/1 -> clutch disengaged/2
  [launch_flag] -> Logical Operator/1
  clutch disengaged/1 -> Logical Operator/2
  Logical Operator/1 -> Switch4/2

== system lib_transmission2/clutch <cl>/clutch model and interface/clutch model/enhancedToWorkspace ==
  In1 : Inport  Port=1  LatchInput=off
  Terminator : Terminator
  wires:
  In1/1 -> Terminator/1

== system lib_transmission2/clutch <cl>/clutch model and interface/clutch model/enhancedToWorkspace1 ==
  In1 : Inport  Port=1  LatchInput=off
  Terminator : Terminator
  wires:
  In1/1 -> Terminator/1

== system lib_transmission2/clutch <cl>/clutch model and interface/clutch model/enhancedToWorkspace2 ==
  In1 : Inport  Port=1  LatchInput=off
  Terminator : Terminator
  wires:
  In1/1 -> Terminator/1

== system lib_transmission2/clutch <cl>/clutch model and interface/clutch model/enhancedToWorkspace3 ==
  In1 : Inport  Port=1  LatchInput=off
  Terminator : Terminator
  wires:
  In1/1 -> Terminator/1

== system lib_transmission2/clutch <cl>/clutch model and interface/clutch model/enhancedToWorkspace4 ==
  In1 : Inport  Port=1  LatchInput=off
  Terminator : Terminator
  wires:
  In1/1 -> Terminator/1

== system lib_transmission2/clutch <cl>/clutch model and interface/clutch model/enhancedToWorkspace5 ==
  In1 : Inport  Port=1  LatchInput=off
  Terminator : Terminator
  wires:
  In1/1 -> Terminator/1

== system lib_transmission2/clutch <cl>/clutch model and interface/clutch model/enhancedToWorkspace6 ==
  In1 : Inport  Port=1  LatchInput=off
  Terminator : Terminator
  wires:
  In1/1 -> Terminator/1

== system lib_transmission2/clutch <cl>/clutch model and interface/clutch model/enhancedToWorkspace7 ==
  In1 : Inport  Port=1  LatchInput=off
  Terminator : Terminator
  wires:
  In1/1 -> Terminator/1

== system lib_transmission2/clutch <cl>/clutch model and interface/clutch model/enhancedToWorkspace8 ==
  In1 : Inport  Port=1  LatchInput=off
  Terminator : Terminator
  wires:
  In1/1 -> Terminator/1

== system lib_transmission2/clutch <cl>/clutch model and interface/clutch model/enhancedToWorkspace9 ==
  In1 : Inport  Port=1  LatchInput=off
  Terminator : Terminator
  wires:
  In1/1 -> Terminator/1

== system lib_transmission2/clutch <cl>/clutch model and interface/clutch model/help ==

== system lib_transmission2/final drive <fd>/model&interface/model/Block NOTES ==
  note: This final drive model includes loss data, rotational inertia, and a gear reduction.
  note: The loss torque is zero when the gears are not turning,
      | and is applied at the input side of the gear reduction.
  note: The inertia torque is the input torque required to accelerate the
      | final drive's inertia as measured on the input side.

== system lib_transmission2/final drive <fd>/model&interface/model/effect of inertia (Nm) ==
  note: The inertia torque is the input torque required to accelerate the
      | final drive's inertia as measured on the input side.
  fd input speed (rad/s) : Inport  Port=1  LatchInput=off
  Gain : Gain  Gain=fd_inertia  Multiplication=Element-wise(K.*u)  SaturateOnIntegerOverflow=on
  d/dt : Derivative
  drag torque (Nm) : Outport  Port=1  InitialOutput=0
  wires:
  Gain/1 -> drag torque (Nm)/1
  d/dt/1 -> Gain/1
  fd input speed (rad/s)/1 -> d/dt/1

== system lib_transmission2/final drive <fd>/model&interface/model/enhancedToWorkspace ==
  In1 : Inport  Port=1  LatchInput=off
  To Workspace : ToWorkspace  VariableName=fd_trq_in_a  SampleTime=-1  SaveFormat=Array
  wires:
  In1/1 -> To Workspace/1

== system lib_transmission2/final drive <fd>/model&interface/model/enhancedToWorkspace1 ==
  In1 : Inport  Port=1  LatchInput=off
  To Workspace : ToWorkspace  VariableName=fd_spd_in_a  SampleTime=-1  SaveFormat=Array
  wires:
  In1/1 -> To Workspace/1

== system lib_transmission2/final drive <fd>/model&interface/model/enhancedToWorkspace2 ==
  In1 : Inport  Port=1  LatchInput=off
  To Workspace : ToWorkspace  VariableName=fd_spd_out_a  SampleTime=-1  SaveFormat=Array
  wires:
  In1/1 -> To Workspace/1

== system lib_transmission2/final drive <fd>/model&interface/model/enhancedToWorkspace3 ==
  In1 : Inport  Port=1  LatchInput=off
  To Workspace : ToWorkspace  VariableName=fd_trq_out_a  SampleTime=-1  SaveFormat=Array
  wires:
  In1/1 -> To Workspace/1

== system lib_transmission2/final drive <fd>/model&interface/model/enhancedToWorkspace4 ==
  In1 : Inport  Port=1  LatchInput=off
  To Workspace : ToWorkspace  VariableName=fd_spd_in_r  SampleTime=-1  SaveFormat=Array
  wires:
  In1/1 -> To Workspace/1

== system lib_transmission2/final drive <fd>/model&interface/model/enhancedToWorkspace5 ==
  In1 : Inport  Port=1  LatchInput=off
  To Workspace : ToWorkspace  VariableName=fd_trq_in_r  SampleTime=-1  SaveFormat=Array
  wires:
  In1/1 -> To Workspace/1

== system lib_transmission2/final drive <fd>/model&interface/model/enhancedToWorkspace6 ==
  In1 : Inport  Port=1  LatchInput=off
  To Workspace : ToWorkspace  VariableName=fd_trq_out_r  SampleTime=-1  SaveFormat=Array
  wires:
  In1/1 -> To Workspace/1

== system lib_transmission2/final drive <fd>/model&interface/model/enhancedToWorkspace7 ==
  In1 : Inport  Port=1  LatchInput=off
  To Workspace : ToWorkspace  VariableName=fd_spd_out_r  SampleTime=-1  SaveFormat=Array
  wires:
  In1/1 -> To Workspace/1

== system lib_transmission2/final drive <fd>/model&interface/model/help ==

== system lib_transmission2/final drive <fd>/model&interface/model/loss (Nm) ==
  note: The loss torque is zero when the gears are not turning,
      | and is applied at the input side of the gear reduction.
  fd output speed (rad/s) : Inport  Port=1  LatchInput=off
  Constant : Constant  Orientation=up  Value=0
  Switch : Switch  Threshold=eps
  final drive loss torque (Nm) : Constant  Value=fd_loss
  drag torque (Nm) : Outport  Port=1  InitialOutput=0
  wires:
  final drive loss torque (Nm)/1 -> Switch/1
  Switch/1 -> drag torque (Nm)/1
  fd output speed (rad/s)/1 -> Switch/2
  Constant/1 -> Switch/3

== system lib_transmission2/gearbox <gb>/gearbox model & interface/gearbox model/Block NOTES ==
  note: This gearbox model includes loss data, rotational inertia, and a gear reduction.
  note: The loss torque is zero when the gears are not turning,
      | and is applied at the input side of the gear reduction.
  note: The inertia torque is the input torque required to accelerate the
      | final drive's inertia as measured on the input side.
  note: Available output torque is estimated assuming that the gearbox efficiency for theavailable input
      | torque andspeed is the same as the gearbox efficiency for the REQUESTED input torque.
  note: This is a good assumption, at least for the VW 4-speed manual transaxle of SAE 820741.
      | In the VW transaxle, efficiency is fairly independent of torque and speed at high torques.
